simulink model "Model2"  (R2020b)
settings: Solver=VariableStepAuto  StartTime=0.0  StopTime=10  RelTol=1e-3
settings Model: Creator=IR13  LastModifiedBy=IR13

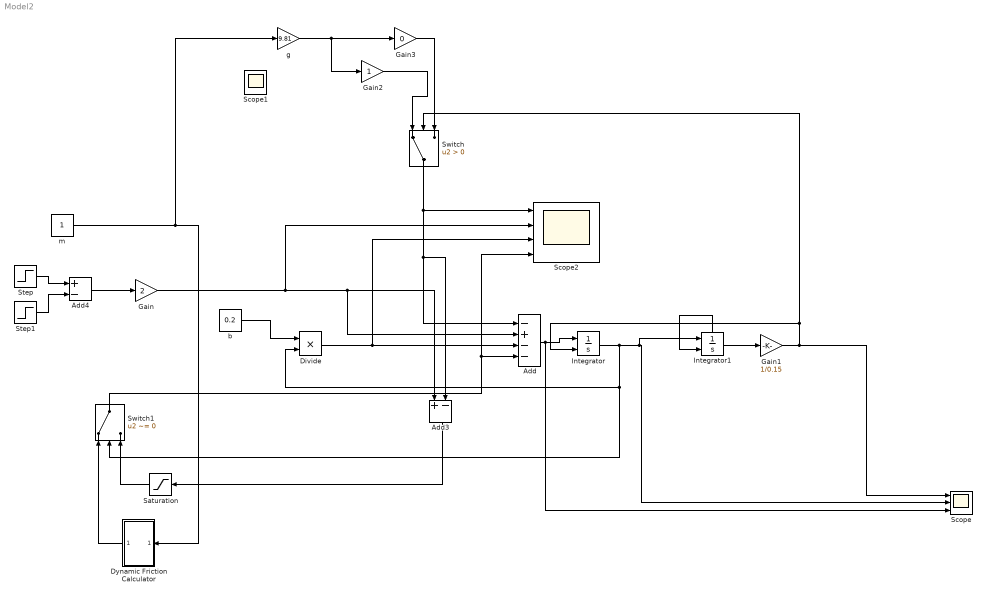
== system Model2 ==
  Add : Sum  Inputs=-+--
  Add3 : Sum  Inputs=+-
  Add4 : Sum  Inputs=+-
  Divide : Product  Inputs=**
  Dynamic Friction Calculator : Subsystem
  Gain : Gain  Gain=2
  Gain1 : Gain  Gain=1/0.15
  Gain2 : Gain
  Gain3 : Gain  Gain=0
  Integrator : Integrator  ExternalReset=falling
  Integrator1 : Integrator  ExternalReset=falling  ShowStatePort=on
  Saturation : Saturate  UpperLimit=0.13*9.81  LowerLimit=-0.13*9.81
  Scope : Scope  NumInputPorts=3
  Scope2 : Scope  NumInputPorts=4
  Step : Step  Time=2  After=10  SampleTime=0
  Step1 : Step  Time=3  After=10  SampleTime=0
  Switch : Switch  Criteria=u2 > Threshold
  Switch1 : Switch  Criteria=u2 ~= 0
  b : Constant  Value=0.2
  g : Gain  Gain=9.81
  m : Constant
  Scope1 : Scope
  wires:
  Gain/1 -> Add/2, Add3/1, Scope2/2
  g/1 -> Gain3/1, Gain2/1
  Integrator/1 -> Switch1/2, Divide/2, Scope/2, Integrator1/1
  Integrator1/1 -> Gain1/1
  b/1 -> Divide/1
  Switch1/1 -> Scope2/4, Add/4
  Step/1 -> Add4/1
  Switch/1 -> Add/1, Add3/2, Scope2/1
  Gain1/1 -> Switch/2, Integrator/2, Scope/1
  Add3/1 -> Saturation/1
  Step1/1 -> Add4/2
  Divide/1 -> Scope2/3, Add/3
  Add/1 -> Scope/3, Integrator/1
  Integrator1/State -> Integrator1/2
  Gain2/1 -> Switch/1
  Gain3/1 -> Switch/3
  m/1 -> Dynamic Friction Calculator/1(In1), g/1
  Dynamic Friction Calculator/1(Out1) -> Switch1/1
  Saturation/1 -> Switch1/3
  Add4/1 -> Gain/1

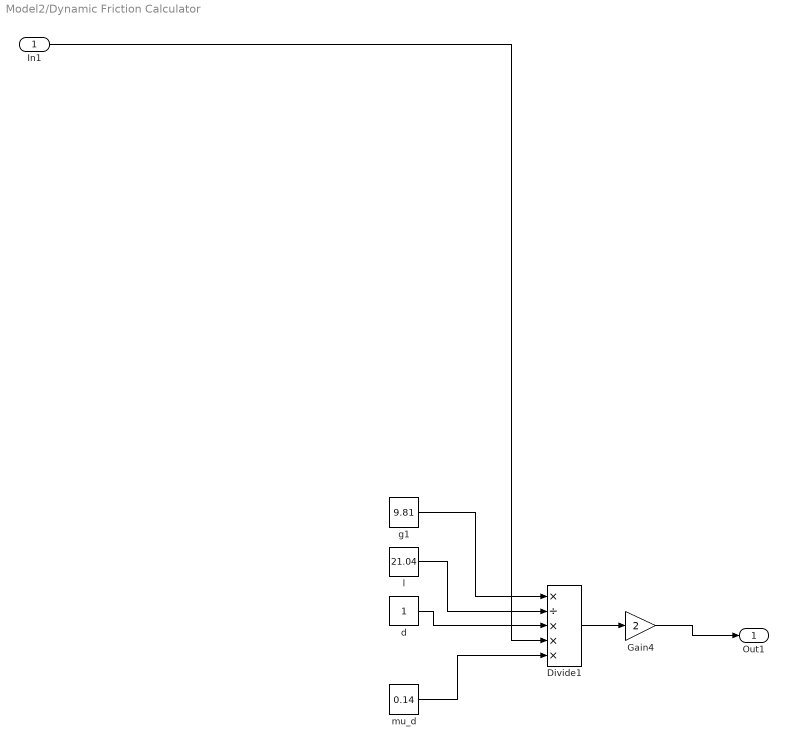
== system Model2/Dynamic Friction Calculator ==
  In1 : Inport
  Divide1 : Product  Inputs=*/***
  Gain4 : Gain  Gain=2
  d : Constant
  g1 : Constant  Value=9.81
  l : Constant  Value=21.04
  mu_d : Constant  Value=0.14
  Out1 : Outport
  wires:
  g1/1 -> Divide1/1
  In1/1 -> Divide1/4
  mu_d/1 -> Divide1/5
  d/1 -> Divide1/3
  Gain4/1 -> Out1/1
  Divide1/1 -> Gain4/1
  l/1 -> Divide1/2
